simulink model "PID_Loop_2023a"  (R2023a)
settings: Solver=FixedStepAuto  StartTime=0.0  StopTime=tspan  FixedStep=dt  RelTol=1e-3
model workspace (MAT data in the model file):
  Drag_Constants = 1
  mass = [5.51 5.51 5.51 1 1 1]
  mass_6a = [5 5 5 1 1 1]
values from neighbouring files (symbols this model uses):
  do_bouyancy_flag = 1    [PID_testing_data_producer.m]    (also in init.m = 0)
  do_drag_flag = 1    [PID_testing_data_producer.m]
  do_gravity_flag = 1    [PID_testing_data_producer.m]    (also in init.m = 0)
  drag_wrench = [ ... (first row only)    [constants.m]    (also in constants.mat = [0.41 0 0 0 0 0 0 0.5 0 0 0 0 ... (36 elements, 6x6)])
  dt = 0.001    [PID_testing_data_producer.m]    (also in init.m)
  Dt = 0.01    [init.m]
  dt_controller = 0.01    [PID_testing_data_producer.m]
  dt_filter = 0.01    [PID_testing_data_producer.m]    (also in init.m)
  dt_imu = 0.01    [PID_testing_data_producer.m]
  dt_plotting = 0.01    [PID_testing_data_producer.m]
  g = 9.8067    [constants.m]    (also in constants.mat = 9.80665)
  H = [1 0 0 ... (first row only)    [init.m]
  inverse_wrench = pinv(wrench)    [calculate_wrench.m]    (also in constants.m = geometry_properties.inverse_wrench; geometry_properties.mat = [0.09 0.09 -0.09 -0.09 0.353553390593 0.353553390593 0.35355)
  max_pitch_torque = norm(wrench*(F_max*[1 1 -1 -1 0 0 0 0]'))    [calculate_wrench.m]
  max_roll_torque = norm(wrench*(F_max*[1 -1 1 -1 0 0 0 0]'))    [calculate_wrench.m]
  max_yaw_torque = norm(wrench*(F_max*[0 0 0 0 -1 1 -1 1]'))    [calculate_wrench.m]
  OperatingVoltage = Voltage    (= 16)    [constants.m]
  Q = diag([0.0001, 0.0001, 0.1])    [init.m]
  R = [.1 0 ... (first row only)    [init.m]
  states_desired = [x_des;E_des]    [init.m]
  v0_e = [0,0,0]'    [PID_testing_data_producer.m]    (also in init.m = [pi/6, -pi/6, pi]')
  Voltage = 16    [constants.m]
  volume = 0.0074    [constants.m]    (also in constants.mat = 0.0073741788)
  volume_center = [0, 0, -0.07]    [constants.m]    (also in constants.mat = [0 0 0.1])
  water_density = 997    [constants.m]    (also in constants.mat = 1000)
  waypoints = input_state_errors(:,i)    [PID_testing_data_producer.m]    (also in init.m = [0, 0, 0])
  wrench = eval(w)    [calculate_wrench.m]    (also in constants.m = geometry_properties.wrench; constants.mat = [0 0 0 0 -0.7071 -0.7071 -0.7071 -0.7071 0 0 0 0 ... (48 ele; geometry_properties.mat = [0 0 -1 0.22 0.25 0 0 0 -1 -0.22 0.25 0 ... (48 elements, 6x; wrench.m)
  x0_e = [0,0,0]'    [PID_testing_data_producer.m]    (also in init.m = [0, 0, 0]')
undefined symbols (not defined in the file or in its folder): IMU, P, Zero_Time
libraries: slpidlib x4, shared6dof x1, mspfiltlib x1, dspstat3 x1, mspsensorlib x1
(part 2 of 2)

== matlab function PID_Loop_2023a/Plant/Gravity and Hydrostatics/Bouyant Force ==
  data: DCMbe input; buoyant_force output; g parameter; water_density parameter; volume parameter; volume_center parameter
function buoyant_force = buoyant_force(DCMbe, g, water_density, volume, volume_center)

    % Ensure d is a column vector
    volume_center = volume_center(:);

    % Buoyant force vector in world frame
    b_vector = [0; 0; water_density * -g * volume];

    % Rotate buoyant force to object's frame
    buoyant_force_body = DCMbe * b_vector;

    % Compute torque using cross product τ = d × F_buoyancy
    % (MATLAB cross function works for column vectors)
    torque = cross(volume_center, buoyant_force_body);

    % Combine force and torque into a single output vector
    buoyant_force = [buoyant_force_body; torque];
end

== matlab function PID_Loop_2023a/Plant/Gravity and Hydrostatics/Weight ==
  data: DCMbe input; weight_force output; g parameter; P parameter; g_b output
function [weight_force,g_b] = weight_force(DCMbe, g, P)
    m = P.m;

    % Gravity force vector in world frame (downward)
    g_vector = [0; 0; m * g];
    
    % Linear Force
    lin = DCMbe * g_vector;
    g_b = DCMbe * [0;0;g];
    % Rotational force
    rot = [0;0;0];
    % Transform gravity force to rotated frame
    weight_force = [lin; rot];
end

== matlab function PID_Loop_2023a/Waypoint Follower/Desired State Generator ==
  data: current_waypoint output; waypoints input; desired_states output; states_des input; current_waypoint_index output; current_waypoint_index input; intermediate_waypoint input; tol parameter; intermediate_waypoint output
function [current_waypoint,desired_states,current_waypoint_index,intermediate_waypoint]= fcn(waypoints,states_des,current_waypoint_index,intermediate_waypoint,tol)

%The initial value of the current_waypoint_index is 1, as set in the data
%store memory block.
x_e = states_des(1:3);

% check the next waypoint in the list
current_waypoint = waypoints(:,current_waypoint_index);

%get the length of the waypoint list
[~, N_wp] = size(waypoints);
% get the position vector to the current waypoint
r_b2wp_e = current_waypoint - x_e;
%get the range to the current waypoint
R_wp = norm(r_b2wp_e);

% get the range to the current intermediate waypoint
r_b2iwp_e = intermediate_waypoint - x_e;
R_int_wp = norm(r_b2iwp_e);

% if the range to the intermediate waypoint is smaller than the tolerance
if(R_wp <= tol)
    %if there is another waypoint on the list, switch the current waypoint
    %to that
    if(current_waypoint_index < N_wp)
        current_waypoint_index = current_waypoint_index + 1; %update wp index
        current_waypoint = waypoints(:,current_waypoint_index); %update wp
    else
        %keep using the current waypoint without changing it
        current_waypoint_index = N_wp;
        current_waypoint = current_waypoint; 
    end
    %recalculate the range
    r_b2wp_e = current_waypoint - x_e;
    R_wp = norm(r_b2wp_e);
end

%if the range to the waypoint and intermediate waypoint is larger than 1
if(R_wp > 1 && R_int_wp > 1)
    %create an intermediate waypoint
    intermediate_waypoint = x_e + r_b2wp_e/R_wp;
    r_b2iwp_e = intermediate_waypoint - x_e;
    R_int_wp = norm(r_b2iwp_e);

%if the range to the waypoint is greater than 1 but the vehicle is close
%the intermediate waypoint 
elseif(R_wp > 1 && R_int_wp <= 1 && R_int_wp > tol)
    %keep using the intermediate waypoint
    intermediate_waypoint = intermediate_waypoint;

%if the vehicle is far from the current waypoint but has reached the
%intermediate waypoint
elseif(R_wp > 1 && R_int_wp <= tol)
    %generate a new intermediate waypoint
    intermediate_waypoint = x_e + r_b2wp_e/R_wp;

%if the vehicle is close to the final waypoint, make the intermediate
%waypoint the final waypoint
elseif(R_wp <= 1)
    intermediate_waypoint = current_waypoint;

else
    %this shouldn't be reached, but here just in case
    intermediate_waypoint = current_waypoint;
end

%bearing angle
E = states_des(4:6); %unpack the euler angles
DCMbe = eul2rotm(E'); %calculate the rotation matrix
r_b2iwp_b = DCMbe*r_b2iwp_e; %calculate the bearing vector in the body frame
%xy_r_b2iwp_b = [r_b2iwp_b(1); r_b2iwp_b(2); 0]; %project onto xy plane

%to do: figure this out
yaw = atan2(r_b2iwp_b(1),r_b2iwp_b(2));

%put on interval -pi to pi
if (yaw > pi)
    yaw = yaw - 2*pi;
end

desired_states = [intermediate_waypoint;[0 0 yaw]'];

end

== matlab function PID_Loop_2023a/Attitude EKF/Euler EKF ==
  data: phi_meas input; theta_meas input; phi_hat output; w_meas input; xhat_prior input; P_prior input; theta_hat output; psi_hat output; dt parameter; H parameter; x output; P output; Q parameter; R parameter
function [phi_hat, theta_hat, psi_hat, x, P] = fcn(phi_meas,theta_meas,w_meas,xhat_prior,P_prior,dt, H, Q, R)

%Inputs: 
%   z = [phi_meas, theta_meas]', the measured euler angles
%   w = [p q r]' the measured angular rates
%   dt = timestep

%changed variable names to match source material
z = [phi_meas, theta_meas]';
x = xhat_prior;
rates = w_meas;
P = P_prior;

A = Ajacob(x, rates, dt); %get state transition matrix from linearization

%Predict
xp = fx(x, rates, dt); %use state transition function to get a priori update of states
Pp = A*P*A' + Q; %compute a priori error covariance matrix

K = Pp*H'*inv(H*Pp*H' + R); %compute kalman gain

%Correct using measurements
x = xp + K*(z - H*xp);
P = Pp - K*H*Pp;

%use built in matlab functions to make sure euler angles are in the correct
%domain
eul = [x(1) x(2) x(3)];
rotmZXY = eul2rotm(eul);
eul = rotm2eul(rotmZXY);

%outputs
phi_hat = eul(1);
theta_hat = eul(2);
psi_hat = eul(3);
x = [phi_hat;theta_hat;psi_hat];



%state transition function
function xp = fx(xhat,rates,dt)
    phi = xhat(1);
    theta = xhat(2);

    p = rates(1);
    q = rates(2);
    r = rates(3);

    xdot = zeros(3,1);

    %euler angle kinematics
    xdot(1) = p + q*sin(phi)*tan(theta) + r*cos(phi)*tan(theta);
    xdot(2) = q*cos(phi) - r*sin(phi);
    xdot(3) = q*sin(phi)*sec(theta) + r*cos(phi)*sec(theta);

    xp = xhat + xdot*dt;

end

%jacobian function
function A = Ajacob(xhat, rates, dt)
    A = zeros(3,3);

    phi = xhat(1);
    theta = xhat(2);

    p = rates(1);
    q = rates(2);
    r = rates(3);

    A(1,1) = q*cos(phi)*tan(theta) - r*sin(phi)*tan(theta);
    A(1,2) = q*sin(phi)*sec(theta)^2 - r*cos(phi)*sec(theta)^2;
    A(1,3) = 0;

    A(2,1) = -q*sin(phi) - r*cos(phi);
    A(2,2) = 0;
    A(2,3) = 0;

    A(3,1) = q*cos(phi)*sec(theta) - r*sin(phi)*sec(theta);
    A(3,2) = q*sin(phi)*sec(theta)*tan(theta) + r*cos(phi)*sec(theta)*tan(theta);
    A(3,3) = 0;

    A = eye(3) + A*dt;
end
end
